simulink model "systemMechanicalFriction"  (R2023b)
settings: Solver=ode45  StartTime=0.0  StopTime=T_SIM  RelTol=1e-3
values from neighbouring files (symbols this model uses):
  spr_traj = 4    [simSpringMassSystem.m]
  X_MAX = 1    [simSpringMassSystem.m]
undefined symbols (not defined in the file or in its folder): parControl, parSys
libraries: simulink x3
settings Model: Creator=GurtnerM  LastModifiedBy=WesthauserP
settings SolverCC: AlgebraicLoopSolver=TrustRegion
settings DataIOCC: ReturnWorkspaceOutputs=off
settings DebuggingCC: UnconnectedInputMsg=warning  UnconnectedOutputMsg=warning  UnconnectedLineMsg=warning  ArithmeticOperatorsInVariantConditions=warning
settings ModelReferenceCC: EnableRefExpFcnMdlSchedulingChecks=on
settings SFSimCC: SimUseLocalCustomCode=off  CustomCodeUndefinedFunction=UseInterfaceOnly
settings RTWCC: RTWUseLocalCustomCode=off  DLArmComputeVersion=19.05

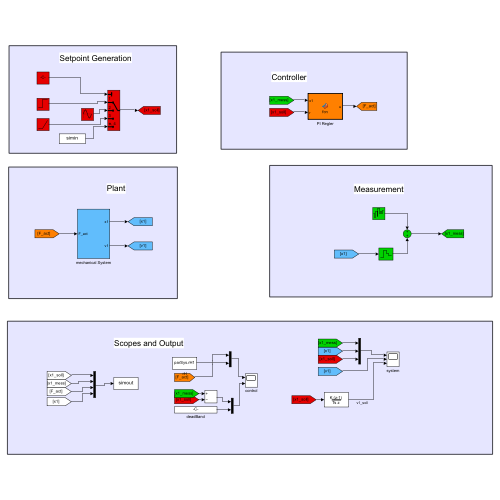
[thumbnail: Simulink's stored preview of the top-level diagram]
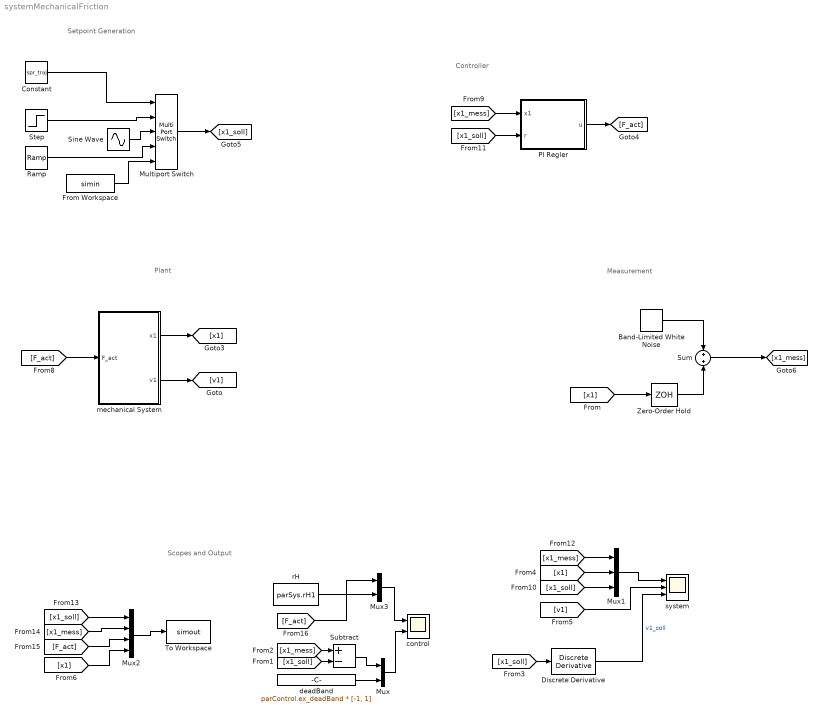
== system systemMechanicalFriction ==
  note: Scopes and Output
  note: Plant
  note: Controller
  note: Measurement
  note: Setpoint Generation
  Band-Limited White Noise : simulink/Sources/Band-Limited White Noise  Cov=1e-8  Ts=parControl.Ts  seed=[23341]
  Constant : Constant  Value=spr_traj
  Discrete Derivative : simulink/Discrete/Discrete Derivative  gainval=1.0  ICPrevScaledInput=0.0  OutMin=[]  OutMax=[]  OutDataType=fixdt(1, 16)  OutScaling=2^-10  DoSatur=off
  From Workspace : FromWorkspace  VariableName=simin
  Multiport Switch : MultiPortSwitch  Inputs=4  SaturateOnIntegerOverflow=off  InputSameDT=off
  Mux : Mux  Inputs=2
  Mux1 : Mux  Inputs=3
  Mux2 : Mux
  Mux3 : Mux  Inputs=2
  PI Regler : MATLAB Function  TreatAsAtomicUnit=on
  Ramp : simulink/Sources/Ramp  slope=0.02/60  start=0  InitialOutput=0.2
  Sine Wave : Sin  Amplitude=0.01  Bias=0.2  Frequency=2*pi/100 * 2  SampleTime=0
  Step : Step  After=X_MAX  SampleTime=0
  Subtract : Sum  Inputs=+-
  Sum : Sum
  To Workspace : ToWorkspace  VariableName=simout  SaveFormat=Structure With Time  SampleTime=parControl.Ts
  Zero-Order Hold : ZeroOrderHold  SampleTime=parControl.Ts
  control : Scope  NumInputPorts=2
  deadBand : Constant  Value=parControl.ex_deadBand * [-1, 1]
  mechanical System : Subsystem
  rH : Constant  Value=parSys.rH1
  system : Scope  NumInputPorts=3
  wires:
  [x1_soll] -> PI Regler/2(r)
  Mux1/1 -> system/1
  [v1] -> system/2
  PI Regler/1(u) -> [F_act]
  [x1_mess] -> PI Regler/1(x1)
  Sum/1 -> [x1_mess]
  Band-Limited White Noise/1 -> Sum/1
  [x1_mess] -> Mux1/1
  [x1] -> Mux1/2
  [x1_soll] -> Mux1/3
  Sine Wave/1 -> Multiport Switch/3
  Ramp/1 -> Multiport Switch/4
  [x1_mess] -> Mux2/2
  [x1_soll] -> Mux2/1
  [F_act] -> Mux2/3
  Mux2/1 -> To Workspace/1
  Multiport Switch/1 -> [x1_soll]
  Constant/1 -> Multiport Switch/1
  Step/1 -> Multiport Switch/2
  Zero-Order Hold/1 -> Sum/2
  [x1] -> Zero-Order Hold/1
  [F_act] -> mechanical System/1(F_act)
  mechanical System/1(x1) -> [x1]
  mechanical System/2(v1) -> [v1]
  [x1_mess] -> Subtract/1
  [x1_soll] -> Subtract/2
  Subtract/1 -> Mux/1
  deadBand/1 -> Mux/2
  Mux/1 -> control/2
  [x1_soll] -> Discrete Derivative/1
  Discrete Derivative/1 -> system/3  "v1_soll"
  From Workspace/1 -> Multiport Switch/5
  [x1] -> Mux2/4
  [F_act] -> Mux3/1
  Mux3/1 -> control/1
  rH/1 -> Mux3/2

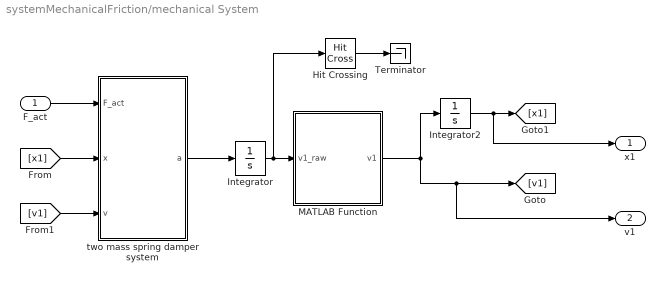
== system systemMechanicalFriction/mechanical System ==
  F_act : Inport
  Hit Crossing : HitCross
  Integrator : Integrator
  Integrator2 : Integrator  InitialCondition=parSys.x1_0
  MATLAB Function : MATLAB Function  TreatAsAtomicUnit=on
  Terminator : Terminator
  two mass spring damper system : MATLAB Function  TreatAsAtomicUnit=on
  x1 : Outport
  v1 : Outport  Port=2
  wires:
  Hit Crossing/1 -> Terminator/1
  F_act/1 -> two mass spring damper system/1(F_act)
  [x1] -> two mass spring damper system/2(x)
  Integrator2/1 -> x1/1, [x1]
  two mass spring damper system/1(a) -> Integrator/1
  [v1] -> two mass spring damper system/3(v)
  MATLAB Function/1(v1) -> v1/1, [v1], Integrator2/1
  Integrator/1 -> MATLAB Function/1(v1_raw), Hit Crossing/1

== matlab function systemMechanicalFriction/PI Regler ==
  settings: updateMethod=DISCRETE  sampleTime=parControl.Ts
  data: x1 input; u output; r input; parControl parameter
function u = fcn(x1, r, parControl)

persistent eI

if isempty(eI)
    eI = 0;
end

kp = parControl.kp;
kI = parControl.kI;
Ta = parControl.Ts;
ex_tol = parControl.ex_deadBand;
u_max = parControl.u_max;

e_raw = x1-r;

switch parControl.controlType
    case 'deadZone'
        e = limitedError(e_raw, ex_tol);    % i.e. Dead Zone
        eI = eI + e * Ta;
        u = -kp * e - kI *eI;

    case 'freeze'
        e = e_raw;
        if abs(e) > ex_tol
            eI = eI + e * Ta;
        end
        u = -kp * e - kI *eI;
        
    otherwise
        u = 0; e = 0;   % to stop matlab from complaining :) 
end

if abs(u) > u_max
    u = u_max * sign(u);
    eI = eI - e * Ta;
end

end
% ------------------------------------------

function e = limitedError(eRaw, eTol)
eAbs = abs(eRaw);
if eAbs < eTol
    e = 0;
else
    e = (eAbs - eTol) * sign(eRaw);
end
end

== matlab function systemMechanicalFriction/mechanical System/two mass spring damper system ==
  data: F_act input; a output; x input; v input; parSys parameter
function a = fcn(F_act, x, v, parSys)

% F_act ... actuation force on mass
% x ... postion of mass 
% v ... velocity of mass

% |   c1
% |--/\/\--|-----|
% |   d1   | m1  |---->F_act2
% |----|---|-----|
% |         x1,v1
    
    p = parSys;
    m = p.m1;
    c = p.c1;
    rv = p.rv;
    x1_0 = p.x1_0;
    v0 = p.v0;

    v_th = p.vStuck;
    
    rH = p.rH1;
    rC = p.rC1;
    
    F1 = -c * (x-x1_0) + F_act;
    
    % m stuck:
    if abs(v) < v_th && abs(F1) < rH
        a = 0;
    else   
        Fr = rv * v + rC*sign(v) + (rH - rC) * exp(-(v/v0)^2) * sign(v); 
        a = 1/m * (F1 - Fr);
    end

end

== matlab function systemMechanicalFriction/mechanical System/MATLAB Function ==
  data: v1_raw input; v1 output; parSys parameter
function v1  = fcn(v1_raw, parSys)
    
    v_th = parSys.vStuck;
    
    if abs(v1_raw) < v_th
        v1 = 0;
    else
        v1 = v1_raw;
    end

end
